simulink model "motor_position_ctr"  (R2020a)
settings: Solver=ode45  StartTime=0.0  StopTime=10.0  RelTol=1e-3
model workspace (MAT data in the model file):
  J = 3.2284e-06
  K = 0.0274
  L = 2.75e-06
  R = 4
  b = 3.5077e-06
settings Model: DataDictionary=prob4.sldd  Creator=HP  LastModifiedBy=HP

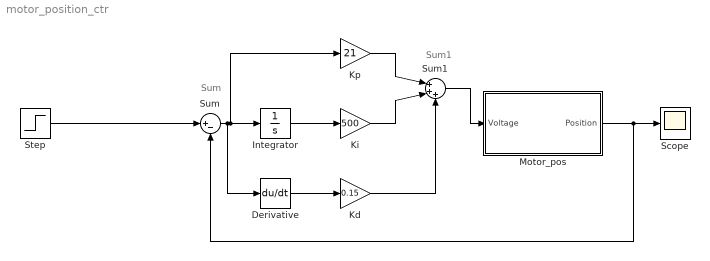
== system motor_position_ctr ==
  note: Sum1
  note: Sum
  Derivative : Derivative
  Integrator : Integrator
  Kd : Gain  Gain=0.15
  Ki : Gain  Gain=500
  Kp : Gain  Gain=21
  Motor_pos : Subsystem
  Scope : Scope
  Step : Step  SampleTime=0
  Sum : Sum  Inputs=|+-
  Sum1 : Sum  Inputs=|+++
  wires:
  Derivative/1 -> Kd/1
  Kd/1 -> Sum1/3
  Ki/1 -> Sum1/2
  Integrator/1 -> Ki/1
  Kp/1 -> Sum1/1
  Sum/1 -> Derivative/1, Kp/1, Integrator/1
  Sum1/1 -> Motor_pos/1(Voltage)
  Step/1 -> Sum/1
  Motor_pos/1(Position) -> Sum/2, Scope/1

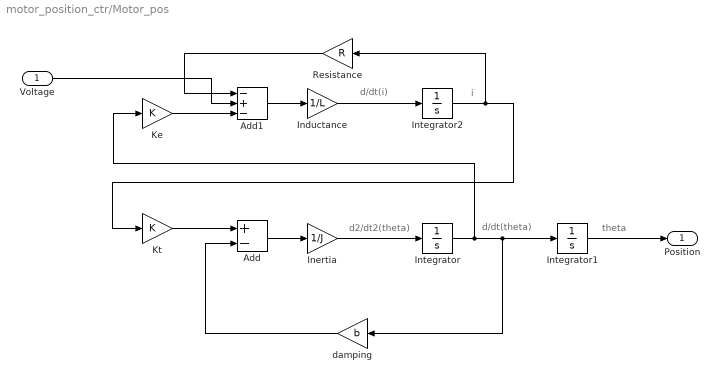
== system motor_position_ctr/Motor_pos ==
  note: i
  note: d/dt(i)
  note: d2/dt2(theta)
  note: d/dt(theta)
  note: theta
  Voltage : Inport
  Add : Sum  Inputs=+-
  Add1 : Sum  Inputs=-+-
  Inductance : Gain  Gain=1/L
  Inertia : Gain  Gain=1/J
  Integrator : Integrator
  Integrator1 : Integrator
  Integrator2 : Integrator
  Ke : Gain  Gain=K
  Kt : Gain  Gain=K
  Resistance : Gain  Gain=R
  damping : Gain  Gain=b
  Position : Outport
  wires:
  Inertia/1 -> Integrator/1
  Inductance/1 -> Integrator2/1
  Integrator2/1 -> Resistance/1, Kt/1
  Integrator/1 -> Ke/1, damping/1, Integrator1/1
  Integrator1/1 -> Position/1
  Voltage/1 -> Add1/2
  Add/1 -> Inertia/1
  damping/1 -> Add/2
  Kt/1 -> Add/1
  Resistance/1 -> Add1/1
  Ke/1 -> Add1/3
  Add1/1 -> Inductance/1
